simulink model "Finger_Full_Model"  (Simulink 8.3)
settings: Solver=ode4  StartTime=0.0  StopTime=20  FixedStep=0.001  RelTol=1e-7
values from neighbouring files (symbols this model uses):
  bCM = 0.035    [Initialization.m]
  Cp = 322.0    (= 322)    [Initialization.m]
  Da = 75.0e9    (= 75000000000)    [Initialization.m]
  Dm = 28.0e9    (= 28000000000)    [Initialization.m]
  Dw = 375.0e-6    (= 0.000375)    [Initialization.m]
  eps0_1 = dX1/Lw1    (= 0.0218549084951)    [Initialization.m]
  eps0_2 = dX2/Lw2    (= 0.016675268755)    [Initialization.m]
  epsR1 = 0.023    [Initialization.m]
  epsR2 = 0.023    [Initialization.m]
  g = 9.81    [Initialization.m]
  Inertia = 4.88e-5    (= 4.88e-05)    [Initialization.m]
  m = 1.5e-2    (= 0.015)    [Initialization.m]
  Mw = dens*pi*(Dw^2)/4    (= 0.000712380677894)    [Initialization.m]
  Rw = 8.66    [Initialization.m]
  Sw = pi*Dw^2/4    (= 1.10446616728e-07)    [Initialization.m]
  Tamb = 60    [Initialization.m]
  theta0 = -40*(pi/180)    (= -0.698131700798)    [Initialization.m]
  thetaT = 0    [Initialization.m]
  vel0 = 0*(pi/180)    (= 0)    [Initialization.m]
settings Model: Creator=GabGil  LastModifiedBy=GabGil  ExtModeArmWhenConnect=off  BufferReuse=off
settings SolverCC: AlgebraicLoopSolver=LineSearch
settings OptimizationCC: BlockReduction=off  BooleanDataType=off  OptimizeBlockIOStorage=off  BufferReuse=off  GlobalBufferReuse=off  ExpressionFolding=off  LocalBlockOutputs=off  InitFltsAndDblsToZero=on
settings DebuggingCC: AlgebraicLoopMsg=none  SaveWithParameterizedLinksMsg=none  SignalResolutionControl=TryResolveAllWithWarning  MultiTaskDSMMsg=warning  MultiTaskCondExecSysMsg=none  FrameProcessingCompatibilityMsg=error  StateNameClashWarn=none
settings RTWCC: SystemTargetFile=wincon.tlc  MakeCommand=make_wc  TemplateMakefile=wc_default_tmf  Description=WinCon Target  ProcessScript=wincon_make_rtw_hook
settings STFCustomTargetCC: TargetFcnLib=ansi_tfl_tmw.mat  ModelReferenceCompliant=off  CPPClassGenCompliant=on  SystemTargetFile=wincon.tlc
settings GRTTargetCC: TargetFcnLib=ansi_tfl_tmw.mat  ModelReferenceCompliant=off  ParMdlRefBuildCompliant=off  CompOptLevelCompliant=off  ConcurrentExecutionCompliant=off  GeneratePreprocessorConditionals=Use local settings  MatFileLogging=off  ExtMode=on  ExtModeTransport=2  ExtModeMexFile=wc_comm
settings CustomProperty: Value=on
settings ConfigComp: CovMetricSettings=dw  CovHtmlReporting=on  CovSaveCumulativeToWorkspaceVar=on  CovSaveSingleToWorkspaceVar=on  CovExternalEMLEnable=off

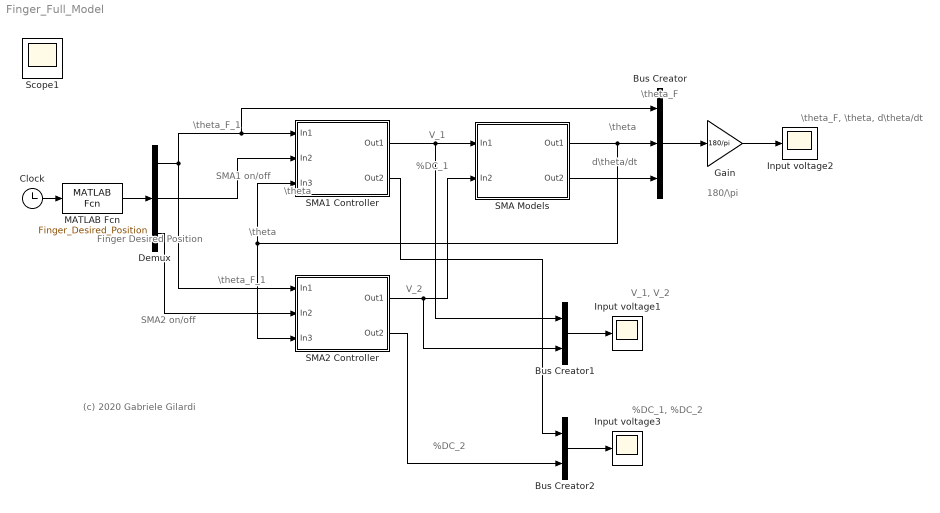
== system Finger_Full_Model ==
  note: (c) 2020 Gabriele Gilardi
  note: 180/\pi
  note: \theta_F_1
  note: \theta_F, \theta, d\theta/dt
  note: \theta
  note: \theta
  note: V_1
  note: V_2
  note: d\theta/dt
  note: \theta_F
  note: V_1, V_2
  note: %DC_1, %DC_2
  note: Finger Desired
      | Position
  note: SMA1
      | on/off
  note: SMA2
      | on/off
  note: \theta
  note: %DC_1
  note: %DC_2
  note: \theta_F_1
  Bus Creator : BusCreator  DialogController=Simulink.DDGSource_Bus  Inputs=3
  Bus Creator1 : BusCreator  DialogController=Simulink.DDGSource_Bus  Inputs=2
  Bus Creator2 : BusCreator  DialogController=Simulink.DDGSource_Bus  Inputs=2
  Clock : Clock
  Demux : Demux  Outputs=[1 1 1]
  Gain : Gain  Gain=180/pi
  Input voltage1 : Scope
      settings: SaveName=V_time
  Input voltage2 : Scope
      settings: YMin=-40  YMax=25  SaveName=theta_time
  Input voltage3 : Scope
      settings: SaveName=pDC_time
  MATLAB Fcn : MATLABFcn  MATLABFcn=Finger_Desired_Position  OutputDimensions=3
  SMA Models : Subsystem
  SMA1 Controller : Subsystem
  SMA2 Controller : Subsystem
  Scope1 : Scope
  wires:
  SMA1 Controller/1(Out1) -> SMA Models/1(In1), Bus Creator1/1
  SMA Models/1(Out1) -> SMA1 Controller/3(In3), SMA2 Controller/3(In3), Bus Creator/2
  SMA Models/2(Out2) -> Bus Creator/3
  Bus Creator/1 -> Gain/1
  Gain/1 -> Input voltage2/1
  Clock/1 -> MATLAB Fcn/1
  Bus Creator1/1 -> Input voltage1/1
  SMA2 Controller/1(Out1) -> SMA Models/2(In2), Bus Creator1/2
  Bus Creator2/1 -> Input voltage3/1
  SMA2 Controller/2(Out2) -> Bus Creator2/2
  SMA1 Controller/2(Out2) -> Bus Creator2/1
  MATLAB Fcn/1 -> Demux/1
  Demux/1 -> SMA2 Controller/1(In1), Bus Creator/1, SMA1 Controller/1(In1)
  Demux/2 -> SMA1 Controller/2(In2)
  Demux/3 -> SMA2 Controller/2(In2)

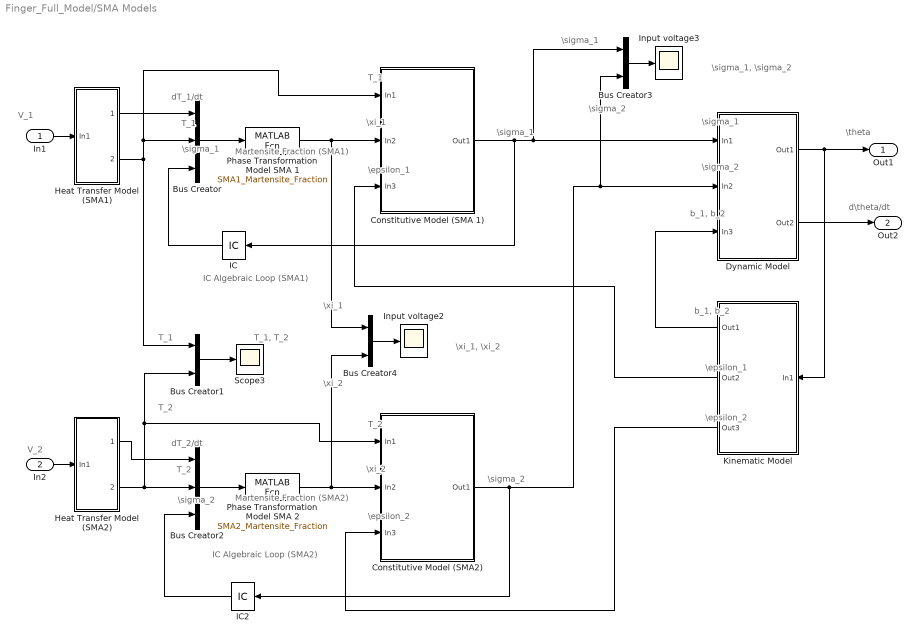
== system Finger_Full_Model/SMA Models ==
  note: IC Algebraic
      | Loop (SMA1)
  note: Martensite
      | Fraction (SMA1)
  note: T_1
  note: \xi_1
  note: dT_1/dt
  note: \sigma_1
  note: \epsilon_1
  note: \theta
  note: d\theta/dt
  note: \xi_1, \xi_2
  note: \sigma_1, \sigma_2
  note: T_1, T_2
  note: V_1
  note: \sigma_1
  note: \epsilon_1
  note: T_2
  note: \xi_2
  note: dT_2/dt
  note: \sigma_2
  note: \epsilon_2
  note: V_2
  note: \sigma_2
  note: \epsilon_2
  note: \sigma_2
  note: b_1, b_2
  note: T_1
  note: T_2
  note: \sigma_1
  note: b_1, b_2
  note: T_1
  note: T_2
  note: \sigma_1
  note: \sigma_2
  note: \xi_1
  note: \xi_2
  note: Martensite
      | Fraction (SMA2)
  note: IC Algebraic
      | Loop (SMA2)
  In1 : Inport
  In2 : Inport  Port=2
  Bus Creator : BusCreator  DialogController=Simulink.DDGSource_Bus  Inputs=3
  Bus Creator1 : BusCreator  DialogController=Simulink.DDGSource_Bus  Inputs=2
  Bus Creator2 : BusCreator  DialogController=Simulink.DDGSource_Bus  Inputs=3
  Bus Creator3 : BusCreator  DialogController=Simulink.DDGSource_Bus  Inputs=2
  Bus Creator4 : BusCreator  DialogController=Simulink.DDGSource_Bus  Inputs=2
  Constitutive Model (SMA 1) : Subsystem
  Constitutive Model (SMA2) : Subsystem
  Dynamic Model : Subsystem
  Heat Transfer Model (SMA1) : Subsystem
  Heat Transfer Model (SMA2) : Subsystem
  IC : InitialCondition  Value=0
  IC2 : InitialCondition  Value=0
  Input voltage2 : Scope
      settings: SaveName=xi_time
  Input voltage3 : Scope
      settings: SaveName=sigma_time
  Kinematic Model : Subsystem
  Phase Transformation Model SMA 1 : MATLABFcn  MATLABFcn=SMA1_Martensite_Fraction  OutputDimensions=1
  Phase Transformation Model SMA 2 : MATLABFcn  MATLABFcn=SMA2_Martensite_Fraction  OutputDimensions=1
  Scope3 : Scope
      settings: SaveName=T_time  MaxDataPoints=50000
  Out1 : Outport
  Out2 : Outport  Port=2
  wires:
  In1/1 -> Heat Transfer Model (SMA1)/1(In1)
  Heat Transfer Model (SMA1)/2(Out2) -> Bus Creator1/1, Bus Creator/2, Constitutive Model (SMA 1)/1(In1)
  Heat Transfer Model (SMA1)/1(Out1) -> Bus Creator/1
  Phase Transformation Model SMA 1/1 -> Constitutive Model (SMA 1)/2(In2), Bus Creator4/1
  Bus Creator/1 -> Phase Transformation Model SMA 1/1
  Bus Creator1/1 -> Scope3/1
  In2/1 -> Heat Transfer Model (SMA2)/1(In1)
  Heat Transfer Model (SMA2)/2(Out2) -> Bus Creator2/2, Bus Creator1/2, Constitutive Model (SMA2)/1(In1)
  Heat Transfer Model (SMA2)/1(Out1) -> Bus Creator2/1
  Constitutive Model (SMA2)/1(Out1) -> IC2/1, Dynamic Model/2(In2), Bus Creator3/2
  Phase Transformation Model SMA 2/1 -> Bus Creator4/2, Constitutive Model (SMA2)/2(In2)
  Bus Creator2/1 -> Phase Transformation Model SMA 2/1
  Dynamic Model/1(Out1) -> Kinematic Model/1(In1), Out1/1
  Dynamic Model/2(Out2) -> Out2/1
  Bus Creator3/1 -> Input voltage3/1
  Bus Creator4/1 -> Input voltage2/1
  Kinematic Model/3(Out3) -> Constitutive Model (SMA2)/3(In3)
  Kinematic Model/2(Out2) -> Constitutive Model (SMA 1)/3(In3)
  Kinematic Model/1(Out1) -> Dynamic Model/3(In3)
  Constitutive Model (SMA 1)/1(Out1) -> IC/1, Bus Creator3/1, Dynamic Model/1(In1)
  IC2/1 -> Bus Creator2/3
  IC/1 -> Bus Creator/3

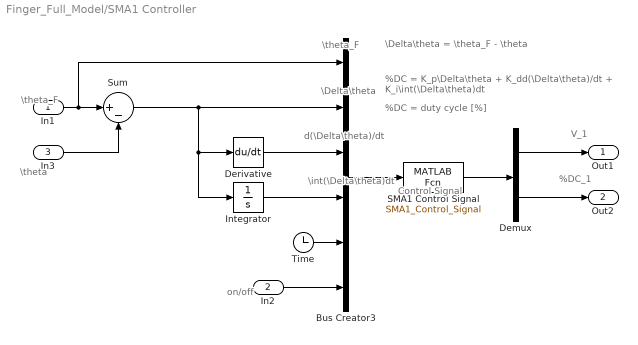
== system Finger_Full_Model/SMA1 Controller ==
  note: Control Signal
  note: \Delta\theta
  note: V_1
  note: \theta_F
  note: \theta
  note: %DC_1
  note: d(\Delta\theta)/dt
  note: \int(\Delta\theta)dt
  note: \theta_F
  note: %DC = duty cycle [%]
  note: %DC = K_p\Delta\theta + K_dd(\Delta\theta)/dt + K_i\int(\Delta\theta)dt
  note: \Delta\theta = \theta_F - \theta
  note: on/off
  In1 : Inport
  In2 : Inport  Port=2
  In3 : Inport  Port=3
  Bus Creator3 : BusCreator  DialogController=Simulink.DDGSource_Bus  Inputs=6
  Demux : Demux  Outputs=[1 1]
  Derivative : Derivative
  Integrator : Integrator
  SMA1 Control Signal : MATLABFcn  MATLABFcn=SMA1_Control_Signal  OutputDimensions=2  Output1D=off
  Sum : Sum  Inputs=|+-
  Time : Clock
  Out1 : Outport
  Out2 : Outport  Port=2
  wires:
  In1/1 -> Bus Creator3/1, Sum/1
  Demux/1 -> Out1/1
  Demux/2 -> Out2/1
  Bus Creator3/1 -> SMA1 Control Signal/1
  SMA1 Control Signal/1 -> Demux/1
  Derivative/1 -> Bus Creator3/3
  Time/1 -> Bus Creator3/5
  Integrator/1 -> Bus Creator3/4
  Sum/1 -> Bus Creator3/2, Integrator/1, Derivative/1
  In3/1 -> Sum/2
  In2/1 -> Bus Creator3/6

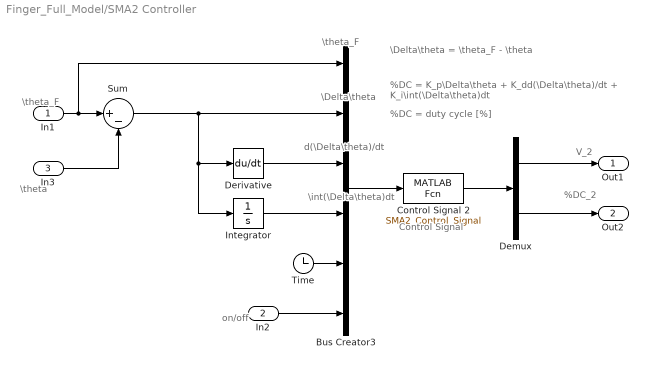
== system Finger_Full_Model/SMA2 Controller ==
  note: Control Signal
  note: \Delta\theta
  note: \theta_F
  note: \theta
  note: %DC_2
  note: d(\Delta\theta)/dt
  note: \int(\Delta\theta)dt
  note: \theta_F
  note: V_2
  note: %DC = duty cycle [%]
  note: %DC = K_p\Delta\theta + K_dd(\Delta\theta)/dt + K_i\int(\Delta\theta)dt
  note: \Delta\theta = \theta_F - \theta
  note: on/off
  In1 : Inport
  In2 : Inport  Port=2
  In3 : Inport  Port=3
  Bus Creator3 : BusCreator  DialogController=Simulink.DDGSource_Bus  Inputs=6
  Control Signal 2 : MATLABFcn  MATLABFcn=SMA2_Control_Signal  OutputDimensions=2  Output1D=off
  Demux : Demux  Outputs=[1 1]
  Derivative : Derivative
  Integrator : Integrator
  Sum : Sum  Inputs=|+-
  Time : Clock
  Out1 : Outport
  Out2 : Outport  Port=2
  wires:
  In1/1 -> Sum/1, Bus Creator3/1
  Demux/1 -> Out1/1
  Demux/2 -> Out2/1
  Bus Creator3/1 -> Control Signal 2/1
  Control Signal 2/1 -> Demux/1
  Derivative/1 -> Bus Creator3/3
  Time/1 -> Bus Creator3/5
  Integrator/1 -> Bus Creator3/4
  Sum/1 -> Bus Creator3/2, Integrator/1, Derivative/1
  In3/1 -> Sum/2
  In2/1 -> Bus Creator3/6

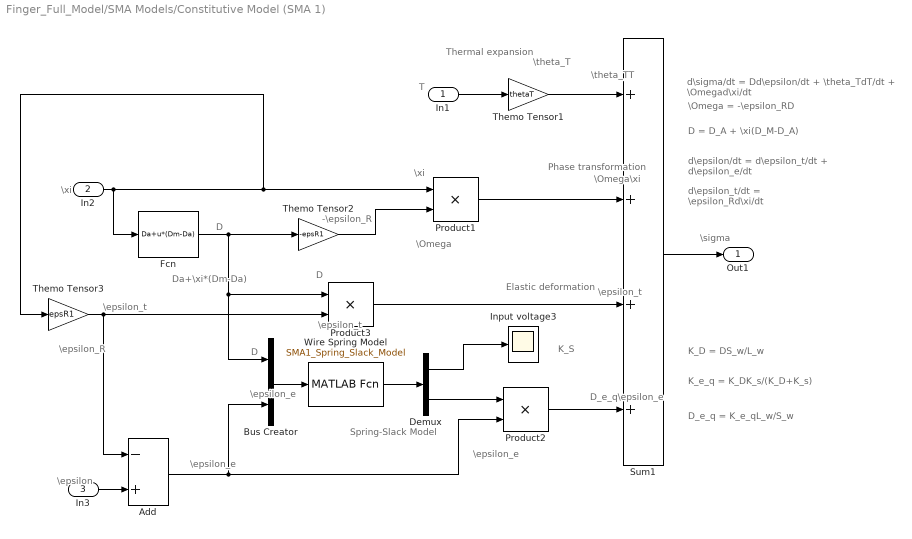
== system Finger_Full_Model/SMA Models/Constitutive Model (SMA 1) ==
  note: \xi
  note: \xi
  note: \Omega = -\epsilon_RD
  note: \theta_T
  note: \theta_TT
  note: \Omega\xi
  note: \sigma
  note: \epsilon
  note: d\sigma/dt = Dd\epsilon/dt + \theta_TdT/dt + \Omegad\xi/dt
  note: T
  note: \Omega
  note: d\epsilon/dt = d\epsilon_t/dt + d\epsilon_e/dt
  note: d\epsilon_t/dt = \epsilon_Rd\xi/dt
  note: -\epsilon_R
  note: D
  note: \epsilon_R
  note: \epsilon_t
  note: \epsilon_e
  note: \epsilon_t
  note: D_e_q\epsilon_e
  note: D = D_A + \xi(D_M-D_A)
  note: K_e_q = K_DK_s/(K_D+K_s)
  note: Thermal expansion
  note: Phase transformation
  note: Da+\xi*(Dm-Da)
  note: Elastic deformation
  note: K_D = DS_w/L_w
  note: K_S
  note: D_e_q = K_e_qL_w/S_w
  note: Spring-Slack
      | Model
  note: \epsilon_e
  note: D
  note: \epsilon_e
  note: D
  note: \epsilon_t
  In1 : Inport
  In2 : Inport  Port=2
  In3 : Inport  Port=3
  Add : Sum  Inputs=-+
  Bus Creator : BusCreator  DialogController=Simulink.DDGSource_Bus  Inputs=2
  Demux : Demux  Outputs=2
  Fcn : Fcn  Expr=Da+u*(Dm-Da)
  Input voltage3 : Scope
      settings: SaveName=Ks1_time
  Product1 : Product  RndMeth=Zero
  Product2 : Product  RndMeth=Zero
  Product3 : Product  RndMeth=Zero
  Sum1 : Sum  Inputs=++++  SaturateOnIntegerOverflow=on
  Themo Tensor1 : Gain  Gain=thetaT  SaturateOnIntegerOverflow=on  OutDataTypeStr=Inherit: Same as input  ParamDataTypeStr=Inherit: Same as input
  Themo Tensor2 : Gain  Gain=-epsR1  SaturateOnIntegerOverflow=on  OutDataTypeStr=Inherit: Same as input  ParamDataTypeStr=Inherit: Same as input
  Themo Tensor3 : Gain  Gain=epsR1  SaturateOnIntegerOverflow=on  OutDataTypeStr=Inherit: Same as input  ParamDataTypeStr=Inherit: Same as input
  Wire Spring Model : MATLABFcn  MATLABFcn=SMA1_Spring_Slack_Model  OutputDimensions=2
  Out1 : Outport
  wires:
  Sum1/1 -> Out1/1
  In1/1 -> Themo Tensor1/1
  In2/1 -> Fcn/1, Product1/1, Themo Tensor3/1
  Themo Tensor3/1 -> Product3/2, Add/1
  In3/1 -> Add/2
  Fcn/1 -> Bus Creator/1, Product3/1, Themo Tensor2/1
  Themo Tensor2/1 -> Product1/2
  Add/1 -> Product2/2, Bus Creator/2
  Bus Creator/1 -> Wire Spring Model/1
  Themo Tensor1/1 -> Sum1/1
  Product3/1 -> Sum1/3
  Product2/1 -> Sum1/4
  Product1/1 -> Sum1/2
  Wire Spring Model/1 -> Demux/1
  Demux/2 -> Product2/1
  Demux/1 -> Input voltage3/1

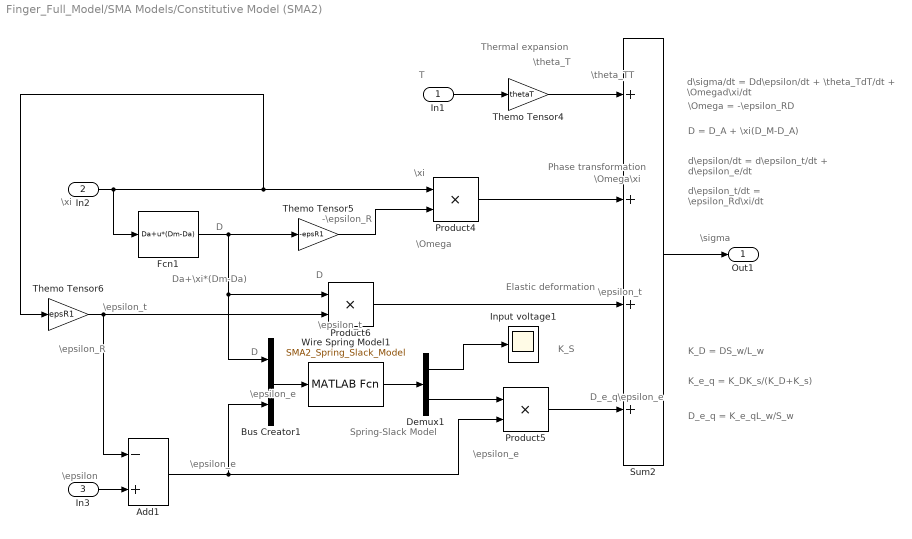
== system Finger_Full_Model/SMA Models/Constitutive Model (SMA2) ==
  note: \xi
  note: \xi
  note: \Omega = -\epsilon_RD
  note: \theta_T
  note: \theta_TT
  note: \Omega\xi
  note: \sigma
  note: \epsilon
  note: d\sigma/dt = Dd\epsilon/dt + \theta_TdT/dt + \Omegad\xi/dt
  note: T
  note: \Omega
  note: d\epsilon/dt = d\epsilon_t/dt + d\epsilon_e/dt
  note: d\epsilon_t/dt = \epsilon_Rd\xi/dt
  note: -\epsilon_R
  note: D
  note: \epsilon_R
  note: \epsilon_t
  note: \epsilon_e
  note: \epsilon_t
  note: D_e_q\epsilon_e
  note: D = D_A + \xi(D_M-D_A)
  note: K_e_q = K_DK_s/(K_D+K_s)
  note: Thermal expansion
  note: Phase transformation
  note: Da+\xi*(Dm-Da)
  note: Elastic deformation
  note: K_D = DS_w/L_w
  note: K_S
  note: D_e_q = K_e_qL_w/S_w
  note: Spring-Slack
      | Model
  note: \epsilon_e
  note: D
  note: \epsilon_e
  note: D
  note: \epsilon_t
  In1 : Inport
  In2 : Inport  Port=2
  In3 : Inport  Port=3
  Add1 : Sum  Inputs=-+
  Bus Creator1 : BusCreator  DialogController=Simulink.DDGSource_Bus  Inputs=2
  Demux1 : Demux  Outputs=2
  Fcn1 : Fcn  Expr=Da+u*(Dm-Da)
  Input voltage1 : Scope
      settings: SaveName=Ks2_time
  Product4 : Product  RndMeth=Zero
  Product5 : Product  RndMeth=Zero
  Product6 : Product  RndMeth=Zero
  Sum2 : Sum  Inputs=++++  SaturateOnIntegerOverflow=on
  Themo Tensor4 : Gain  Gain=thetaT  SaturateOnIntegerOverflow=on  OutDataTypeStr=Inherit: Same as input  ParamDataTypeStr=Inherit: Same as input
  Themo Tensor5 : Gain  Gain=-epsR1  SaturateOnIntegerOverflow=on  OutDataTypeStr=Inherit: Same as input  ParamDataTypeStr=Inherit: Same as input
  Themo Tensor6 : Gain  Gain=epsR1  SaturateOnIntegerOverflow=on  OutDataTypeStr=Inherit: Same as input  ParamDataTypeStr=Inherit: Same as input
  Wire Spring Model1 : MATLABFcn  MATLABFcn=SMA2_Spring_Slack_Model  OutputDimensions=2
  Out1 : Outport
  wires:
  Sum2/1 -> Out1/1
  In1/1 -> Themo Tensor4/1
  In2/1 -> Fcn1/1, Product4/1, Themo Tensor6/1
  Themo Tensor6/1 -> Product6/2, Add1/1
  In3/1 -> Add1/2
  Fcn1/1 -> Bus Creator1/1, Product6/1, Themo Tensor5/1
  Themo Tensor5/1 -> Product4/2
  Add1/1 -> Product5/2, Bus Creator1/2
  Bus Creator1/1 -> Wire Spring Model1/1
  Themo Tensor4/1 -> Sum2/1
  Product6/1 -> Sum2/3
  Product5/1 -> Sum2/4
  Product4/1 -> Sum2/2
  Wire Spring Model1/1 -> Demux1/1
  Demux1/2 -> Product5/1
  Demux1/1 -> Input voltage1/1

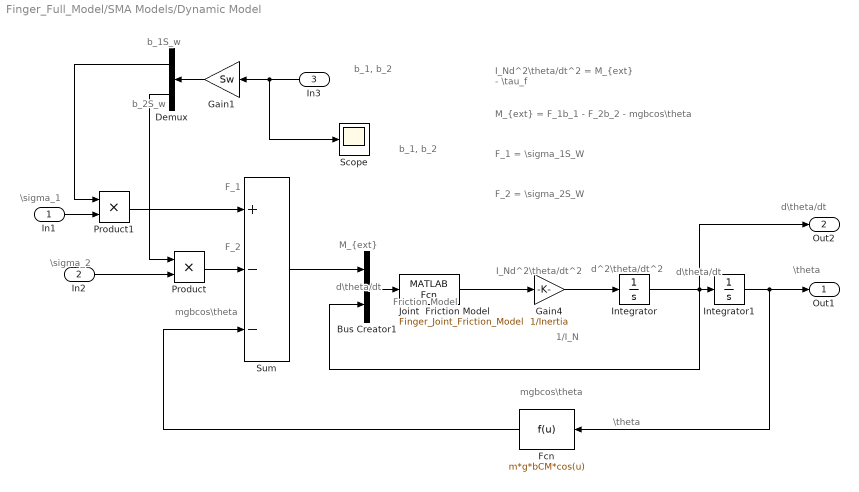
== system Finger_Full_Model/SMA Models/Dynamic Model ==
  note: Friction Model
  note: 1/I_N
  note: d\theta/dt
  note: \theta
  note: d^2\theta/dt^2
  note: I_Nd^2\theta/dt^2
  note: \sigma_1
  note: \theta
  note: d\theta/dt
  note: I_Nd^2\theta/dt^2 = M_{ext} - \tau_f
  note: F_1 = \sigma_1S_W
  note: M_{ext}
  note: d\theta/dt
  note: \sigma_2
  note: F_2 = \sigma_2S_W
  note: M_{ext} = F_1b_1 - F_2b_2 - mgbcos\theta
  note: b_1, b_2
  note: b_1S_w
  note: b_2S_w
  note: F_1
  note: F_2
  note: mgbcos\theta
  note: mgbcos\theta
  note: b_1, b_2
  In1 : Inport
  In2 : Inport  Port=2
  In3 : Inport  Port=3
  Bus Creator1 : BusCreator  DialogController=Simulink.DDGSource_Bus  Inputs=2
  Demux : Demux  Outputs=2
  Fcn : Fcn  Expr=m*g*bCM*cos(u)
  Gain1 : Gain  Gain=Sw  SaturateOnIntegerOverflow=on  OutDataTypeStr=Inherit: Same as input  ParamDataTypeStr=Inherit: Same as input
  Gain4 : Gain  Gain=1/Inertia  SaturateOnIntegerOverflow=on  OutDataTypeStr=Inherit: Same as input  ParamDataTypeStr=Inherit: Same as input
  Integrator : Integrator  InitialCondition=vel0
  Integrator1 : Integrator  InitialCondition=theta0
  Joint  Friction Model : MATLABFcn  MATLABFcn=Finger_Joint_Friction_Model  OutputDimensions=1
  Product : Product  RndMeth=Zero
  Product1 : Product  RndMeth=Zero
  Scope : Scope
      settings: SaveName=b_time
  Sum : Sum  Inputs=+--  SaturateOnIntegerOverflow=on
  Out1 : Outport
  Out2 : Outport  Port=2
  wires:
  Integrator1/1 -> Out1/1, Fcn/1
  Gain4/1 -> Integrator/1
  Product1/1 -> Sum/1
  Fcn/1 -> Sum/3
  Sum/1 -> Bus Creator1/1
  Integrator/1 -> Integrator1/1, Bus Creator1/2, Out2/1
  Bus Creator1/1 -> Joint  Friction Model/1
  Product/1 -> Sum/2
  In1/1 -> Product1/2
  In3/1 -> Gain1/1, Scope/1
  Gain1/1 -> Demux/1
  In2/1 -> Product/2
  Demux/2 -> Product/1
  Demux/1 -> Product1/1
  Joint  Friction Model/1 -> Gain4/1

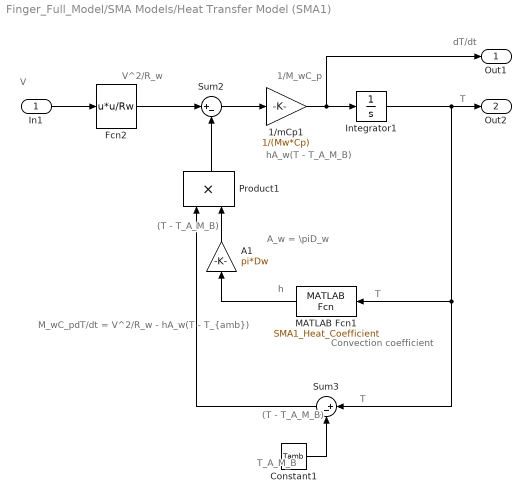
== system Finger_Full_Model/SMA Models/Heat Transfer Model (SMA1) ==
  note: h
  note: A_w = \piD_w
  note: T
  note: M_wC_pdT/dt = V^2/R_w - hA_w(T - T_{amb})
  note: 1/M_wC_p
  note: hA_w(T - T_A_M_B)
  note: V^2/R_w
  note: dT/dt
  note: V
  note: T
  note: T
  note: Convection
      | coefficient
  note: (T - T_A_M_B)
  note: (T - T_A_M_B)
  note: T_A_M_B
  In1 : Inport
  1/mCp1 : Gain  Gain=1/(Mw*Cp)  SaturateOnIntegerOverflow=on  OutDataTypeStr=Inherit: Same as input  ParamDataTypeStr=Inherit: Same as input
  A1 : Gain  Gain=pi*Dw  SaturateOnIntegerOverflow=on  OutDataTypeStr=Inherit: Same as input  ParamDataTypeStr=Inherit: Same as input
  Constant1 : Constant  Value=Tamb
  Fcn2 : Fcn  Expr=u*u/Rw
  Integrator1 : Integrator  InitialCondition=Tamb
  MATLAB Fcn1 : MATLABFcn  MATLABFcn=SMA1_Heat_Coefficient
  Product1 : Product  SaturateOnIntegerOverflow=on  OutDataTypeStr=Inherit: Same as first input
  Sum2 : Sum  Inputs=|+-  SaturateOnIntegerOverflow=on
  Sum3 : Sum  Inputs=|+-  SaturateOnIntegerOverflow=on
  Out1 : Outport
  Out2 : Outport  Port=2
  wires:
  A1/1 -> Product1/2
  Product1/1 -> Sum2/2
  Integrator1/1 -> Out2/1, Sum3/1, MATLAB Fcn1/1
  1/mCp1/1 -> Out1/1, Integrator1/1
  Sum2/1 -> 1/mCp1/1
  Fcn2/1 -> Sum2/1
  Sum3/1 -> Product1/1
  MATLAB Fcn1/1 -> A1/1
  Constant1/1 -> Sum3/2
  In1/1 -> Fcn2/1

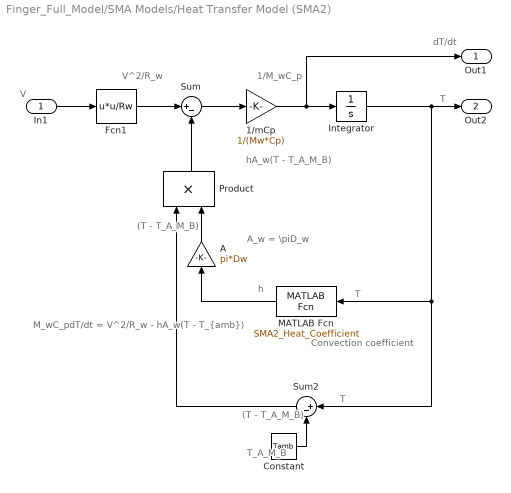
== system Finger_Full_Model/SMA Models/Heat Transfer Model (SMA2) ==
  note: h
  note: A_w = \piD_w
  note: T
  note: M_wC_pdT/dt = V^2/R_w - hA_w(T - T_{amb})
  note: 1/M_wC_p
  note: hA_w(T - T_A_M_B)
  note: V^2/R_w
  note: dT/dt
  note: V
  note: T
  note: T
  note: Convection
      | coefficient
  note: (T - T_A_M_B)
  note: (T - T_A_M_B)
  note: T_A_M_B
  In1 : Inport
  1/mCp : Gain  Gain=1/(Mw*Cp)  SaturateOnIntegerOverflow=on  OutDataTypeStr=Inherit: Same as input  ParamDataTypeStr=Inherit: Same as input
  A : Gain  Gain=pi*Dw  SaturateOnIntegerOverflow=on  OutDataTypeStr=Inherit: Same as input  ParamDataTypeStr=Inherit: Same as input
  Constant : Constant  Value=Tamb
  Fcn1 : Fcn  Expr=u*u/Rw
  Integrator : Integrator  InitialCondition=Tamb
  MATLAB Fcn : MATLABFcn  MATLABFcn=SMA2_Heat_Coefficient
  Product : Product  SaturateOnIntegerOverflow=on  OutDataTypeStr=Inherit: Same as first input
  Sum : Sum  Inputs=|+-  SaturateOnIntegerOverflow=on
  Sum2 : Sum  Inputs=|+-  SaturateOnIntegerOverflow=on
  Out1 : Outport
  Out2 : Outport  Port=2
  wires:
  In1/1 -> Fcn1/1
  A/1 -> Product/2
  Product/1 -> Sum/2
  Integrator/1 -> Out2/1, Sum2/1, MATLAB Fcn/1
  1/mCp/1 -> Out1/1, Integrator/1
  Sum/1 -> 1/mCp/1
  Fcn1/1 -> Sum/1
  Sum2/1 -> Product/1
  MATLAB Fcn/1 -> A/1
  Constant/1 -> Sum2/2

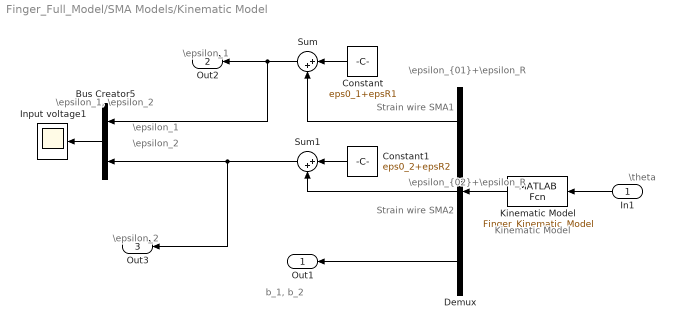
== system Finger_Full_Model/SMA Models/Kinematic Model ==
  note: Kinematic Model
  note: \epsilon_1
  note: \epsilon_1
  note: \epsilon_2
  note: \epsilon_2
  note: \epsilon_1, \epsilon_2
  note: \theta
  note: b_1, b_2
  note: \epsilon_{01}+\epsilon_R
  note: \epsilon_{02}+\epsilon_R
  note: Strain wire SMA1
  note: Strain wire SMA2
  In1 : Inport
  Bus Creator5 : BusCreator  DialogController=Simulink.DDGSource_Bus  Inputs=2
  Constant : Constant  Value=eps0_1+epsR1
  Constant1 : Constant  Value=eps0_2+epsR2
  Demux : Demux  Outputs=[1 1 2]
  Input voltage1 : Scope
      settings: SaveName=eps_time
  Kinematic Model : MATLABFcn  MATLABFcn=Finger_Kinematic_Model  OutputDimensions=4
  Sum : Sum  Inputs=|++
  Sum1 : Sum  Inputs=|++
  Out1 : Outport
  Out2 : Outport  Port=2
  Out3 : Outport  Port=3
  wires:
  Bus Creator5/1 -> Input voltage1/1
  In1/1 -> Kinematic Model/1
  Kinematic Model/1 -> Demux/1
  Demux/3 -> Out1/1
  Constant/1 -> Sum/1
  Demux/1 -> Sum/2
  Sum/1 -> Bus Creator5/1, Out2/1
  Constant1/1 -> Sum1/1
  Demux/2 -> Sum1/2
  Sum1/1 -> Bus Creator5/2, Out3/1
